simulink model "Sinpwmtoankydelay"  (R2022b)
settings: Solver=VariableStepAuto  StartTime=0.0  StopTime=0.03  RelTol=1e-3
libraries: spsOnDelayLib x6, spsIGBTLib x6, simulink x3, spsDCVoltageSourceLib x1, spsGroundLib x1, spsThreePhaseParallelRLCBranchLib x1, spsThreePhaseVIMeasurementLib x1, spsTriangleGeneratorLib x1, spspowerguiLib x1
settings Model: Creator=doand  LastModifiedBy=doand

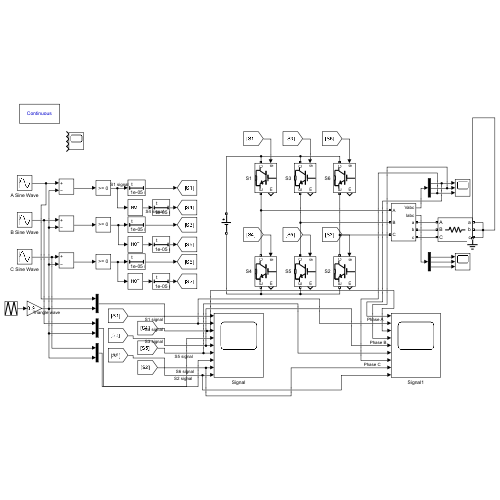
[thumbnail: Simulink's stored preview of the top-level diagram]
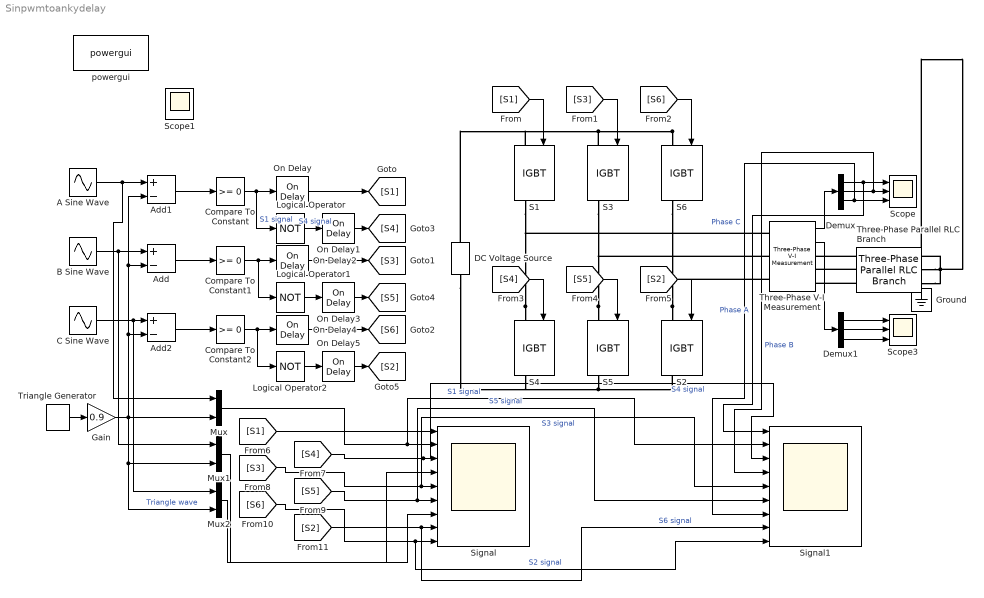
== system Sinpwmtoankydelay ==
  A Sine Wave : Sin  Frequency=2*pi*50  SampleTime=0
  Add : Sum  Inputs=+-
  Add1 : Sum  Inputs=+-
  Add2 : Sum  Inputs=+-
  B Sine Wave : Sin  Frequency=2*pi*50  Phase=2*pi/3  SampleTime=0
  C Sine Wave : Sin  Frequency=2*pi*50  Phase=-2*pi/3  SampleTime=0
  Compare To Constant : simulink/Logic and Bit Operations/Compare To Constant  relop=>=  const=0  OutDataTypeStr=boolean
  Compare To Constant1 : simulink/Logic and Bit Operations/Compare To Constant  relop=>=  const=0  OutDataTypeStr=boolean
  Compare To Constant2 : simulink/Logic and Bit Operations/Compare To Constant  relop=>=  const=0  OutDataTypeStr=boolean
  DC Voltage Source : spsDCVoltageSourceLib/DC Voltage Source  Amplitude=270  Measurements=None
  Demux : Demux  Outputs=3
  Demux1 : Demux  Outputs=3
  Gain : Gain  Gain=0.9
  Ground : spsGroundLib/Ground  LConnTagsString=a
  Logical Operator : Logic  Operator=NOT  AllPortsSameDT=off  OutDataTypeStr=boolean
  Logical Operator1 : Logic  Operator=NOT  AllPortsSameDT=off  OutDataTypeStr=boolean
  Logical Operator2 : Logic  Operator=NOT  AllPortsSameDT=off  OutDataTypeStr=boolean
  Mux : Mux  Inputs=2
  Mux1 : Mux  Inputs=2
  Mux2 : Mux  Inputs=2
  On Delay{,1..5} (6 alike) : spsOnDelayLib/On Delay  DelayType=On delay  delay=0.00001  ic=0  Ts=0
  S{1..6} (6 alike) : spsIGBTLib/IGBT  Ron=0.001  Lon=0  Vf=1  Tf=1e-6  Tt=2e-6  IC=0  Rs=1e5  Cs=inf  Measurements=on
  Scope : Scope  NumInputPorts=3
  Scope1 : Scope  NumInputPorts=4
  Scope3 : Scope  NumInputPorts=3
  Signal : Scope  NumInputPorts=9
  Signal1 : Scope  NumInputPorts=9
  Three-Phase Parallel RLC Branch : spsThreePhaseParallelRLCBranchLib/Three-Phase Parallel RLC Branch  LConnTagsString=A|B|C  RConnTagsString=A|B|C  BranchType=R  Resistance=43  Inductance=1e-3  Capacitance=1e-6  Measurements=Branch voltages and currents
  Three-Phase V-I Measurement : spsThreePhaseVIMeasurementLib/Three-Phase V-I Measurement  VoltageMeasurement=phase-to-phase  SetLabelV=off  LabelV=Vabc  Vpu=off  VpuLL=off  CurrentMeasurement=yes  SetLabelI=off  LabelI=Iabc  Ipu=off  Pbase=100e6  Vbase=500e3  OutputType=Complex  PhasorSimulation=off  PSBequivalent=0
  Triangle Generator : spsTriangleGeneratorLib/Triangle Generator  Freq=2000*4  Phase=0  Ts=0
  powergui : spspowerguiLib/powergui  Priority=1  SimulationMode=Continuous  SampleTime=50e-6  frequency=60  Iterations=50  frequencyindice=0  Pbase=100e6  ErrMax=1e-4  UnitsV=kV  UnitsW=MW  buscounter=0  FunctionMessages=off  echomessages=off  EnableUseOfTLC=off  CurrentSourceSwitches=off  DisableSnubberDevices=off  DisableRonSwitches=off  DisableVfSwitches=off  DisplayEquations=off  AutomaticDiscreteSolvers=off  SolverType=Tustin/Backward Euler (TBE)  Interpol=off  ExternalGateDelay=off  methode=off  Ts=100  x0status=blocks  SPID=on  SwTol=0  HookPort=off  NonlinearTolerance=1e-4  nMaxIteration=100  ContinueOnMaxIteration=off  RestoreLinks=warning  ResistiveCurrentMeasurement=off  Frange=[0:2:500]  Ylog=off  Xlog=on  ShowGrid=off  save=off  variable=ZData  structure=0  ZoomFFT=off  StartTime=0.0  cycles=1  DisplayStyle=1  fundamental=60  FreqAxis=off  MaxFrequency=1000  frequencyindicesteady=1  RmsSteady=1  display=off
  wires:
  [S2] -> S2/1
  Demux1/1 -> Scope3/1
  Triangle Generator/1 -> Gain/1
  [S4] -> S4/1
  [S5] -> S5/1
  [S2] -> Signal1/9, Signal/9  "S2 signal"
  C Sine Wave/1 -> Mux2/1, Add2/1
  [S3] -> Signal1/5, Signal/5  "S3 signal"
  Mux1/1 -> Signal/4
  Mux/1 -> Signal/1
  Logical Operator1/1 -> On Delay3/1
  [S1] -> Signal1/2, Signal/2  "S1 signal"
  Mux2/1 -> Signal/7
  [S6] -> Signal1/8, Signal/8  "S6 signal"
  Demux1/3 -> Scope3/3
  Three-Phase V-I Measurement/2 -> Demux1/1
  Demux/3 -> Signal1/7, Scope/3  "Phase C"
  [S6] -> S6/1
  Add2/1 -> Compare To Constant2/1
  Three-Phase V-I Measurement/1 -> Demux/1
  [S4] -> Signal1/3, Signal/3  "S4 signal"
  Compare To Constant2/1 -> On Delay4/1, Logical Operator2/1
  Add/1 -> Compare To Constant1/1
  [S3] -> S3/1
  Add1/1 -> Compare To Constant/1
  Compare To Constant/1 -> On Delay/1, Logical Operator/1  "S1 signal"
  B Sine Wave/1 -> Mux1/1, Add/1
  [S1] -> S1/1
  Demux/1 -> Signal1/1, Scope/1  "Phase A"
  Gain/1 -> Add2/2, Add/2, Add1/2, Mux2/2, Mux1/2, Mux/2  "Triangle wave"
  [S5] -> Signal1/6, Signal/6  "S5 signal"
  A Sine Wave/1 -> Mux/1, Add1/1
  Demux1/2 -> Scope3/2
  Demux/2 -> Signal1/4, Scope/2  "Phase B"
  On Delay1/1 -> [S4]
  On Delay3/1 -> [S5]
  Logical Operator2/1 -> On Delay5/1
  On Delay5/1 -> [S2]
  On Delay/1 -> [S1]
  On Delay4/1 -> [S6]
  Logical Operator/1 -> On Delay1/1  "S4 signal"
  Compare To Constant1/1 -> On Delay2/1, Logical Operator1/1
  On Delay2/1 -> [S3]
  connections:
  S2/LConn1 -- S6/RConn1 -- Three-Phase V-I Measurement/LConn3
  Three-Phase Parallel RLC Branch/RConn2 -- Three-Phase Parallel RLC Branch/RConn1 -- Three-Phase Parallel RLC Branch/RConn3 -- Ground/LConn1
  S5/LConn1 -- S3/RConn1 -- Three-Phase V-I Measurement/LConn2
  S2/RConn1 -- DC Voltage Source/LConn1 -- S4/RConn1 -- S5/RConn1
  S6/LConn1 -- S3/LConn1 -- DC Voltage Source/RConn1 -- S1/LConn1
  S4/LConn1 -- S1/RConn1 -- Three-Phase V-I Measurement/LConn1
  Three-Phase Parallel RLC Branch/LConn3 -- Three-Phase V-I Measurement/RConn3
  Three-Phase Parallel RLC Branch/LConn2 -- Three-Phase V-I Measurement/RConn2
  Three-Phase Parallel RLC Branch/LConn1 -- Three-Phase V-I Measurement/RConn1
